simulink model "acv_lin"  (R2021a)
settings: Solver=VariableStepAuto  StartTime=0.0  StopTime=20  MaxStep=0.01  RelTol=1e-3
InitFcn:
  | start
values from neighbouring files (symbols this model uses):
  dt = 0.1    [start.m]
  Klqr = -lqr(A,B,Q,R)    [start.m]
  Kmod = -place(A,B,roots)    [start.m]
  kp = 20*[-1 1 -1]    [start.m]
  regime = 6    [start.m]
  x0 = [0;0;0]    [start.m]
  xd = [0;0;10*pi/180]    [start.m]
undefined symbols (not defined in the file or in its folder): Kmpc
settings Model: Creator=Ruslan.Sevostianov  LastModifiedBy=mluser
settings SolverCC: AlgebraicLoopSolver=TrustRegion
settings DataIOCC: ReturnWorkspaceOutputs=off
settings DebuggingCC: SFMachineParentedDataDiag=warning  ArithmeticOperatorsInVariantConditions=warning
settings SFSimCC: CustomCodeUndefinedFunction=UseInterfaceOnly

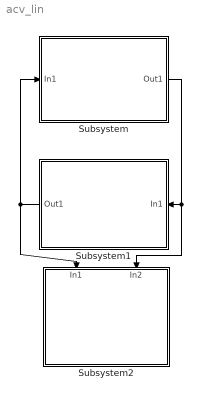
== system acv_lin ==
  Subsystem : Subsystem
      mask Display: disp('Plant')
  Subsystem1 : Subsystem  TreatAsAtomicUnit=on  SystemSampleTime=dt
      mask Display: disp('Control')
  Subsystem2 : Subsystem
      mask Display: disp('Display')
  wires:
  Subsystem/1(Out1) -> Subsystem2/2(In2), Subsystem1/1(In1)
  Subsystem1/1(Out1) -> Subsystem/1(In1), Subsystem2/1(In1)

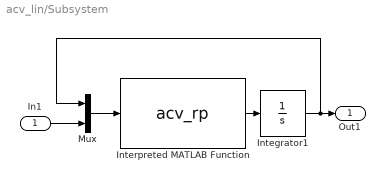
== system acv_lin/Subsystem ==
  In1 : Inport
  Integrator1 : Integrator  InitialCondition=x0
  Interpreted MATLAB Function : MATLABFcn  MATLABFcn=acv_rp  OutputDimensions=3
  Mux : Mux  Inputs=2
  Out1 : Outport  VectorParamsAs1DForOutWhenUnconnected=off
  wires:
  Interpreted MATLAB Function/1 -> Integrator1/1
  Mux/1 -> Interpreted MATLAB Function/1
  In1/1 -> Mux/2
  Integrator1/1 -> Mux/1, Out1/1

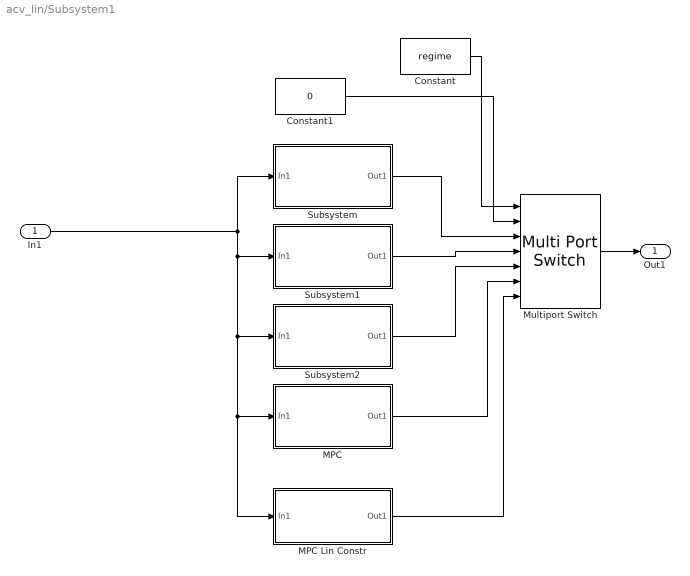
== system acv_lin/Subsystem1 ==
  In1 : Inport
  Constant : Constant  Value=regime
  Constant1 : Constant  Value=0
  MPC : Subsystem
      mask Display: disp('LQR')
  MPC Lin Constr : Subsystem
  Multiport Switch : MultiPortSwitch  Inputs=6
  Subsystem : Subsystem
      mask Display: disp('PID')
  Subsystem1 : Subsystem
      mask Display: disp('Poles')
  Subsystem2 : Subsystem
      mask Display: disp('LQR')
  Out1 : Outport  VectorParamsAs1DForOutWhenUnconnected=off
  wires:
  In1/1 -> MPC Lin Constr/1(In1), MPC/1(In1), Subsystem2/1(In1), Subsystem1/1(In1), Subsystem/1(In1)
  Subsystem/1(Out1) -> Multiport Switch/3
  Subsystem1/1(Out1) -> Multiport Switch/4
  Multiport Switch/1 -> Out1/1
  Constant/1 -> Multiport Switch/1
  Subsystem2/1(Out1) -> Multiport Switch/5
  Constant1/1 -> Multiport Switch/2
  MPC/1(Out1) -> Multiport Switch/6
  MPC Lin Constr/1(Out1) -> Multiport Switch/7

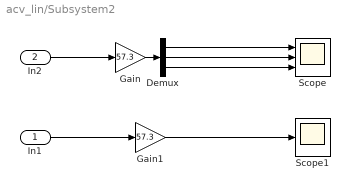
== system acv_lin/Subsystem2 ==
  In1 : Inport
  In2 : Inport  Port=2
  Demux : Demux  Outputs=3
  Gain : Gain  Gain=57.3
  Gain1 : Gain  Gain=57.3
  Scope : Scope  NumInputPorts=3
  Scope1 : Scope
  wires:
  Demux/3 -> Scope/3
  Demux/1 -> Scope/1
  Gain/1 -> Demux/1
  Demux/2 -> Scope/2
  In2/1 -> Gain/1
  In1/1 -> Gain1/1
  Gain1/1 -> Scope1/1

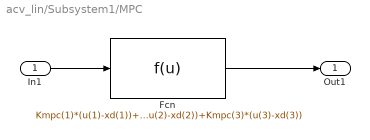
== system acv_lin/Subsystem1/MPC ==
  In1 : Inport
  Fcn : Fcn  Expr=Kmpc(1)*(u(1)-xd(1))+Kmpc(2)*(u(2)-xd(2))+Kmpc(3)*(u(3)-xd(3))
  Out1 : Outport  VectorParamsAs1DForOutWhenUnconnected=off
  wires:
  Fcn/1 -> Out1/1
  In1/1 -> Fcn/1

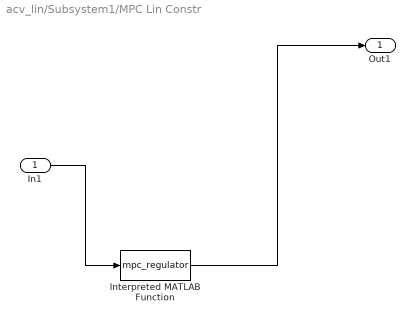
== system acv_lin/Subsystem1/MPC Lin Constr ==
  In1 : Inport
  Interpreted MATLAB Function : MATLABFcn  MATLABFcn=mpc_regulator
  Out1 : Outport
  wires:
  In1/1 -> Interpreted MATLAB Function/1
  Interpreted MATLAB Function/1 -> Out1/1

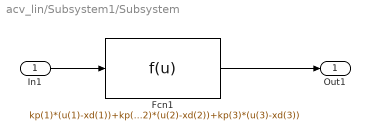
== system acv_lin/Subsystem1/Subsystem ==
  In1 : Inport
  Fcn1 : Fcn  Expr=kp(1)*(u(1)-xd(1))+kp(2)*(u(2)-xd(2))+kp(3)*(u(3)-xd(3))
  Out1 : Outport  VectorParamsAs1DForOutWhenUnconnected=off
  wires:
  Fcn1/1 -> Out1/1
  In1/1 -> Fcn1/1

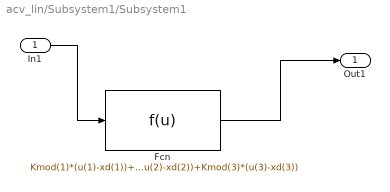
== system acv_lin/Subsystem1/Subsystem1 ==
  In1 : Inport
  Fcn : Fcn  Expr=Kmod(1)*(u(1)-xd(1))+Kmod(2)*(u(2)-xd(2))+Kmod(3)*(u(3)-xd(3))
  Out1 : Outport  VectorParamsAs1DForOutWhenUnconnected=off
  wires:
  Fcn/1 -> Out1/1
  In1/1 -> Fcn/1

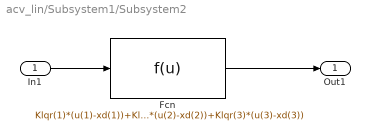
== system acv_lin/Subsystem1/Subsystem2 ==
  In1 : Inport
  Fcn : Fcn  Expr=Klqr(1)*(u(1)-xd(1))+Klqr(2)*(u(2)-xd(2))+Klqr(3)*(u(3)-xd(3))
  Out1 : Outport  VectorParamsAs1DForOutWhenUnconnected=off
  wires:
  Fcn/1 -> Out1/1
  In1/1 -> Fcn/1
